simulink model "sampleModel2085"  (R2023a)
settings: Solver=VariableStepAuto  StartTime=0.0  StopTime=10.0  RelTol=1e-3
libraries: hdlsllib x4, simulink x2
settings Model: Creator=user1  LastModifiedBy=user1

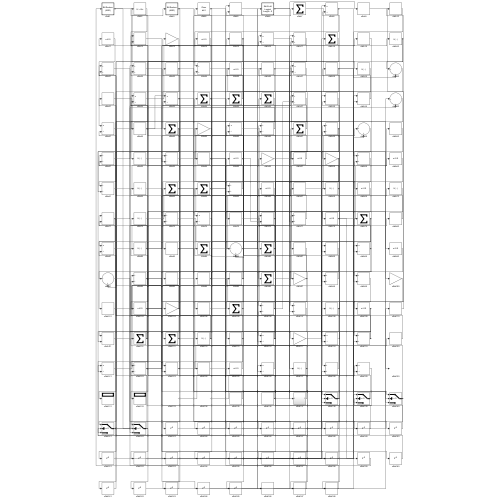
[thumbnail: Simulink's stored preview of the top-level diagram]
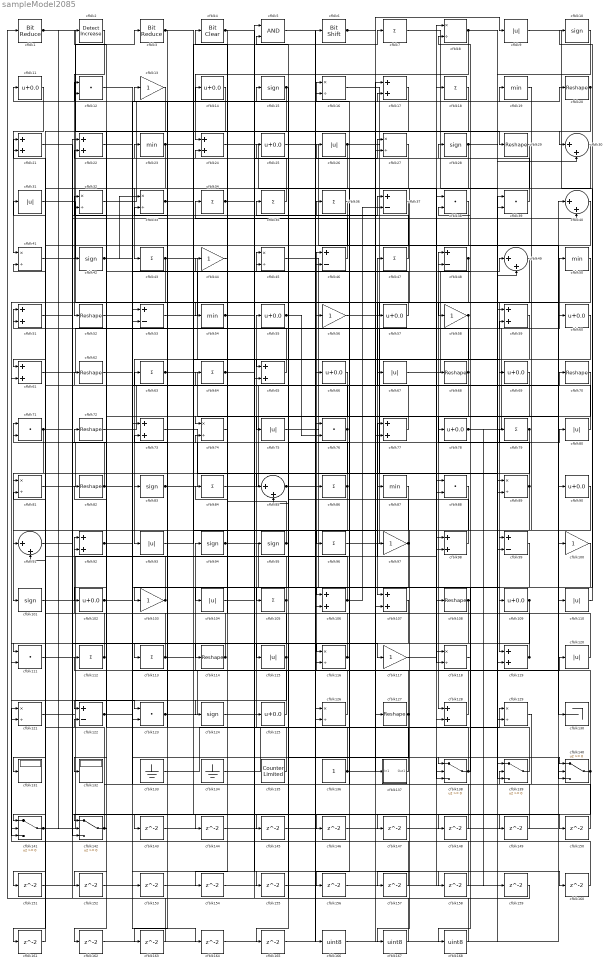
== system sampleModel2085 ==
  cfblk1 : hdlsllib/Logic and Bit Operations/Bit Reduce  mode=AND
  cfblk{10,15,28,42,83,94..95,101,124} (9 alike) : Signum
  cfblk{13,44,56,58,97,100,103,117} (8 alike) : Gain
  cfblk{11,14,25,55,57,60,66,69,78,90,102,109,125} (13 alike) : Bias  Bias=0.0  SaturateOnIntegerOverflow=off
  cfblk{9,26,31,67,75,80,93,104,110,115,120} (11 alike) : Abs  SaturateOnIntegerOverflow=off
  cfblk{7,18,34..36,43,47,63..64,79,84,86,96,105,112..113} (16 alike) : Sum  Inputs=+
  cfblk{17,21..22,24,51,59,61,65,73,77,92,98,106..107,119,128} (16 alike) : Sum
  cfblk{20,29,52,62,68,70,72,82,108,114,127} (11 alike) : Reshape
  cfblk{12,38..39,71,76,88,111,123} (8 alike) : DotProduct  OutDataTypeStr=Inherit: Inherit via internal rule
  cfblk{8,16,27,32..33,41,45,74,81,89,116,118,121,126,129} (15 alike) : Product  Inputs=*/  RndMeth=Zero  SaturateOnIntegerOverflow=on
  cfblk{37,46,48,53,99,122} (6 alike) : Sum  Inputs=+-
  cfblk130 : Terminator
  cfblk131 : Display
  cfblk132 : Display
  cfblk133 : Ground
  cfblk134 : Ground
  cfblk135 : hdlsllib/Sources/Counter Limited  uplimit=7  tsamp=-1
  cfblk136 : Constant  SampleTime=-1
  cfblk137 : Subsystem
      settings: LibrarySourceBlock=|
      | hdlsllib/Ports &
      | Subsystems/Subsystem
  cfblk{138..142} (5 alike) : Switch  SaturateOnIntegerOverflow=off  InputSameDT=off
  cfblk{143..165} (23 alike) : Delay  SampleTime=1
  cfblk166 : DataTypeConversion  OutDataTypeStr=uint8  SaturateOnIntegerOverflow=off  RndMeth=Floor
  cfblk167 : DataTypeConversion  OutDataTypeStr=uint8  SaturateOnIntegerOverflow=off  RndMeth=Floor
  cfblk168 : DataTypeConversion  OutDataTypeStr=uint8  SaturateOnIntegerOverflow=off  RndMeth=Floor
  cfblk{19,23,50,54,87} (5 alike) : MinMax
  cfblk2 : simulink/Logic and Bit Operations/Detect Increase  vinit=0.0  OutDataTypeStr=boolean
      settings: LibrarySourceBlock=|
      | hdlsllib/Logic and Bit
      | Operations/Detect
      | Increase
  cfblk3 : hdlsllib/Logic and Bit Operations/Bit Reduce  mode=AND
  cfblk{30,40,49,85,91} (5 alike) : Sum  Inputs=|++
  cfblk4 : simulink/Logic and Bit Operations/Bit Clear  iBit=0
      settings: LibrarySourceBlock=|
      | hdlsllib/Logic and Bit
      | Operations/Bit Clear
  cfblk5 : Logic  AllPortsSameDT=off  OutDataTypeStr=boolean
  cfblk6 : hdlsllib/Logic and Bit Operations/Bit Shift  mode=Shift Left Logical  N=0
  wires:
  cfblk47/1 -> cfblk35/1
  cfblk114/1 -> cfblk92/1, cfblk73/2
  cfblk41/1 -> cfblk3/1
  cfblk9/1 -> cfblk103/1
  cfblk133/1 -> cfblk129/1
  cfblk49/1 -> cfblk119/1
  cfblk7/1 -> cfblk129/2
  cfblk2/1 -> cfblk52/1
  cfblk134/1 -> cfblk89/1
  cfblk111/1 -> cfblk46/1
  cfblk46/1 -> cfblk34/1
  cfblk45/1 -> cfblk109/1
  cfblk68/1 -> cfblk128/1, cfblk21/2
  cfblk135/1 -> cfblk55/1
  cfblk1/1 -> cfblk29/1, cfblk142/2
  cfblk3/1 -> cfblk97/1, cfblk143/1
  cfblk16/1 -> cfblk89/2
  cfblk67/1 -> cfblk49/1
  cfblk112/1 -> cfblk92/2, cfblk111/1
  cfblk20/1 -> cfblk30/1, cfblk77/2
  cfblk84/1 -> cfblk66/1
  cfblk89/1 -> cfblk48/1, cfblk91/2
  cfblk141/1 -> cfblk68/1, cfblk79/1
  cfblk58/1 -> cfblk93/1, cfblk116/1
  cfblk8/1 -> cfblk24/1, cfblk140/3
  cfblk118/1 -> cfblk28/1
  cfblk43/1 -> cfblk65/1, cfblk61/2, cfblk111/2
  cfblk31/1 -> cfblk130/1
  cfblk97/1 -> cfblk44/1, cfblk116/2
  cfblk120/1 -> cfblk16/1
  cfblk15/1 -> cfblk105/1, cfblk132/1
  cfblk128/1 -> cfblk94/1
  cfblk28/1 -> cfblk59/1, cfblk30/2, cfblk156/1
  cfblk110/1 -> cfblk10/1
  cfblk125/1 -> cfblk112/1
  cfblk80/1 -> cfblk14/1
  cfblk127/1 -> cfblk86/1, cfblk165/1
  cfblk104/1 -> cfblk56/1
  cfblk76/1 -> cfblk101/1, cfblk31/1
  cfblk19/1 -> cfblk99/1
  cfblk27/1 -> cfblk75/1
  cfblk18/1 -> cfblk42/1
  cfblk121/1 -> cfblk123/1
  cfblk82/1 -> cfblk71/1, cfblk45/1, cfblk37/1
  cfblk117/1 -> cfblk18/1
  cfblk140/1 -> cfblk12/2, cfblk152/1
  cfblk56/1 -> cfblk58/1
  cfblk77/1 -> cfblk46/2
  cfblk57/1 -> cfblk2/1
  cfblk102/1 -> cfblk20/1, cfblk138/2, cfblk160/1
  cfblk85/1 -> cfblk70/1, cfblk80/1
  cfblk113/1 -> cfblk71/2, cfblk150/1
  cfblk138/1 -> cfblk32/1, cfblk48/2
  cfblk65/1 -> cfblk22/2
  cfblk48/1 -> cfblk96/1, cfblk91/1
  cfblk142/1 -> cfblk21/1, cfblk162/1
  cfblk115/1 -> cfblk63/1, cfblk121/2
  cfblk71/1 -> cfblk81/1, cfblk36/1
  cfblk38/1 -> cfblk141/1
  cfblk55/1 -> cfblk15/1, cfblk76/2
  cfblk50/1 -> cfblk107/1
  cfblk95/1 -> cfblk4/1, cfblk25/1
  cfblk75/1 -> cfblk98/2
  cfblk69/1 -> cfblk83/1
  cfblk90/1 -> cfblk122/1
  cfblk21/1 -> cfblk117/1
  cfblk106/1 -> cfblk51/1, cfblk37/2
  cfblk61/1 -> cfblk59/2
  cfblk34/1 -> cfblk54/1, cfblk158/1
  cfblk24/1 -> cfblk118/1
  cfblk94/1 -> cfblk137/1(In1), cfblk64/1
  cfblk78/1 -> cfblk50/1, cfblk159/1
  cfblk86/1 -> cfblk123/2, cfblk45/2
  cfblk73/1 -> cfblk85/1
  cfblk11/1 -> cfblk41/1
  cfblk72/1 -> cfblk47/1
  cfblk53/1 -> cfblk39/2
  cfblk137/1(Out1) -> cfblk13/1
  cfblk30/1 -> cfblk57/1
  cfblk4/1 -> cfblk74/1, cfblk87/1
  cfblk64/1 -> cfblk27/1, cfblk138/3
  cfblk17/1 -> cfblk85/2
  cfblk25/1 -> cfblk90/1
  cfblk87/1 -> cfblk107/2
  cfblk10/1 -> cfblk99/2
  cfblk92/1 -> cfblk106/1, cfblk164/1
  cfblk35/1 -> cfblk12/1
  cfblk81/1 -> cfblk74/2
  cfblk13/1 -> cfblk131/1
  cfblk105/1 -> cfblk24/2, cfblk141/3
  cfblk62/1 -> cfblk73/1
  cfblk23/1 -> cfblk69/1, cfblk61/1
  cfblk96/1 -> cfblk60/1
  cfblk26/1 -> cfblk88/2, cfblk104/1
  cfblk63/1 -> cfblk100/1, cfblk33/2, cfblk149/1
  cfblk101/1 -> cfblk77/1
  cfblk51/1 -> cfblk40/2
  cfblk29/1 -> cfblk43/1
  cfblk83/1 -> cfblk17/1, cfblk140/1
  cfblk39/1 -> cfblk26/1
  cfblk119/1 -> cfblk115/1, cfblk84/1
  cfblk42/1 -> cfblk17/2, cfblk33/1
  cfblk66/1 -> cfblk142/1
  cfblk44/1 -> cfblk114/1
  cfblk22/1 -> cfblk53/2
  cfblk98/1 -> cfblk11/1
  cfblk139/1 -> cfblk38/2
  cfblk129/1 -> cfblk139/2
  cfblk126/1 -> cfblk95/1
  cfblk33/1 -> cfblk113/1, cfblk140/2
  cfblk124/1 -> cfblk125/1
  cfblk103/1 -> cfblk32/2, cfblk72/1
  cfblk123/1 -> cfblk108/1, cfblk23/1
  cfblk109/1 -> cfblk142/3, cfblk168/1
  cfblk93/1 -> cfblk7/1
  cfblk54/1 -> cfblk78/1, cfblk138/1
  cfblk32/1 -> cfblk16/2
  cfblk70/1 -> cfblk102/1
  cfblk6/1 -> cfblk127/1, cfblk9/1
  cfblk136/1 -> cfblk82/1, cfblk19/1
  cfblk79/1 -> cfblk118/2, cfblk124/1
  cfblk116/1 -> cfblk76/1, cfblk81/2, cfblk62/1
  cfblk40/1 -> cfblk126/2
  cfblk108/1 -> cfblk8/2, cfblk157/1
  cfblk99/1 -> cfblk139/3
  cfblk122/1 -> cfblk120/1, cfblk67/1
  cfblk143/1 -> cfblk128/2
  cfblk74/1 -> cfblk144/1
  cfblk144/1 -> cfblk65/2
  cfblk107/1 -> cfblk145/1
  cfblk145/1 -> cfblk126/1
  cfblk60/1 -> cfblk146/1
  cfblk146/1 -> cfblk88/1
  cfblk91/1 -> cfblk147/1
  cfblk147/1 -> cfblk40/1
  cfblk100/1 -> cfblk148/1
  cfblk148/1 -> cfblk122/2
  cfblk149/1 -> cfblk106/2
  cfblk150/1 -> cfblk53/1
  cfblk36/1 -> cfblk151/1
  cfblk151/1 -> cfblk139/1
  cfblk152/1 -> cfblk98/1
  cfblk12/1 -> cfblk153/1
  cfblk153/1 -> cfblk38/1
  cfblk59/1 -> cfblk154/1
  cfblk154/1 -> cfblk39/1
  cfblk52/1 -> cfblk155/1
  cfblk155/1 -> cfblk8/1
  cfblk156/1 -> cfblk119/2
  cfblk157/1 -> cfblk141/2
  cfblk158/1 -> cfblk121/1
  cfblk159/1 -> cfblk1/1
  cfblk160/1 -> cfblk41/2
  cfblk14/1 -> cfblk161/1
  cfblk161/1 -> cfblk51/2
  cfblk162/1 -> cfblk49/2
  cfblk37/1 -> cfblk163/1
  cfblk163/1 -> cfblk22/1
  cfblk164/1 -> cfblk27/2
  cfblk165/1 -> cfblk6/1
  cfblk5/1 -> cfblk166/1
  cfblk166/1 -> cfblk110/1
  cfblk88/1 -> cfblk167/1
  cfblk167/1 -> cfblk5/1
  cfblk168/1 -> cfblk5/2

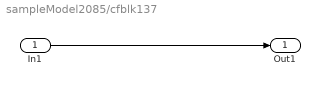
== system sampleModel2085/cfblk137 ==
  In1 : Inport
  Out1 : Outport
  wires:
  In1/1 -> Out1/1
